simulink model "model"  (R2024a)
settings: Solver=FixedStepAuto  StartTime=0.0  StopTime=2500  FixedStep=0.01  RelTol=1e-3
values from neighbouring files (symbols this model uses):
  C_eq1 = [0.99 0 0 0 0 0 0 0 0 0 0 0 ... (924 elements, 22x42)]    [C_1.mat]
  C_eq2 = [0 0 0 0 0 0 0 0 0 0 0 0 ... (22 elements, 22x1)]    [C_2.mat]
  C_ineq1 = [0 0 0 0 0 0 0 0 0 0 0 0 ... (4704 elements, 112x42)]    [C_3.mat]
  C_ineq2 = [0.00443775952052 0.0171604689216 0.00443775952052 0.0171604689216 0.00443775952052 0.0171604689216 0.00443775952052 0.0171604689216 0.00443775952052 0.0171604689216 0.00443775952052 0.0171604689216 ... (112 elements, 112x1)]    [C_4.mat]
  H = [1 0 0 0 0 0 0 0 0 0 0 0 ... (1764 elements, 42x42)]    [H.mat]
settings Model: Creator=12911  LastModifiedBy=12911

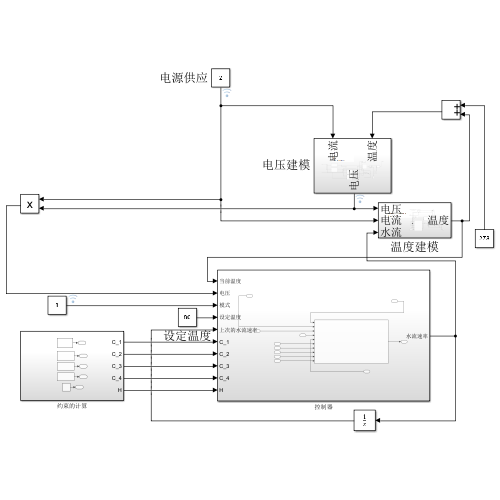
[thumbnail: Simulink's stored preview of the top-level diagram]
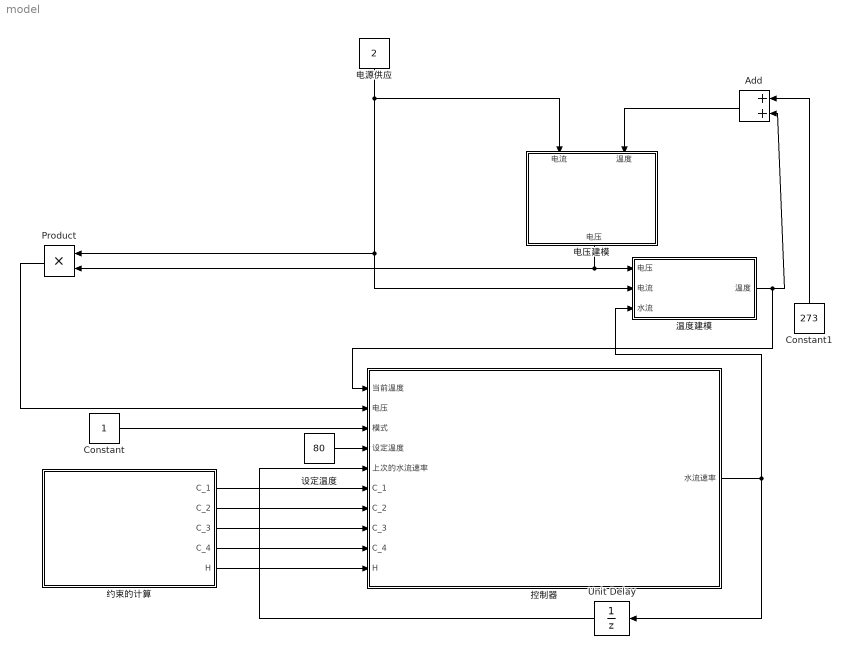
== system model ==
  Add : Sum
  Constant : Constant
  Constant1 : Constant  Value=273
  Product : Product
  Unit Delay : UnitDelay  SampleTime=-1  HasFrameUpgradeWarning=on
  控制器 : Subsystem
  温度建模 : Subsystem
  电压建模 : Subsystem
  电源供应 : Constant  Value=2
  约束的计算 : Subsystem
  设定温度 : Constant  Value=80
  wires:
  电源供应/1 -> 电压建模/1(电流), 温度建模/2(电流), Product/1
  电压建模/1(电压) -> Product/2, 温度建模/1(电压)
  Add/1 -> 电压建模/2(温度)
  Constant1/1 -> Add/1
  温度建模/1(温度) -> 控制器/1(当前温度), Add/2
  控制器/1(水流速率) -> 温度建模/3(水流), Unit Delay/1
  Product/1 -> 控制器/2(电压)
  Constant/1 -> 控制器/3(模式)
  设定温度/1 -> 控制器/4(设定温度)
  Unit Delay/1 -> 控制器/5(上次的水流速率)
  约束的计算/1(C_1) -> 控制器/6(C_1)
  约束的计算/2(C_2) -> 控制器/7(C_2)
  约束的计算/3(C_3) -> 控制器/8(C_3)
  约束的计算/4(C_4) -> 控制器/9(C_4)
  约束的计算/5(H) -> 控制器/10(H)

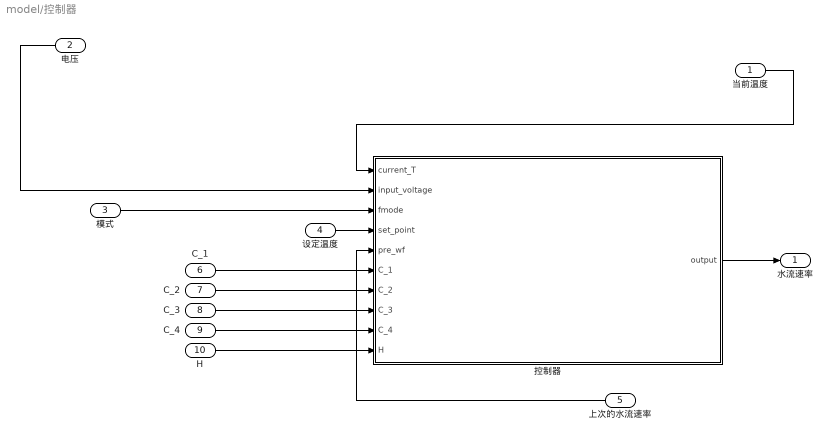
== system model/控制器 ==
  当前温度 : Inport
  电压 : Inport  Port=2
  模式 : Inport  Port=3
  设定温度 : Inport  Port=4
  上次的水流速率 : Inport  Port=5
  C_1 : Inport  Port=6
  C_2 : Inport  Port=7
  C_3 : Inport  Port=8
  C_4 : Inport  Port=9
  H : Inport  Port=10
  控制器 : MATLAB Function  TreatAsAtomicUnit=on
  水流速率 : Outport
  wires:
  当前温度/1 -> 控制器/1(current_T)
  H/1 -> 控制器/10(H)
  C_2/1 -> 控制器/7(C_2)
  模式/1 -> 控制器/3(fmode)
  C_3/1 -> 控制器/8(C_3)
  C_4/1 -> 控制器/9(C_4)
  上次的水流速率/1 -> 控制器/5(pre_wf)
  设定温度/1 -> 控制器/4(set_point)
  控制器/1(output) -> 水流速率/1
  电压/1 -> 控制器/2(input_voltage)
  C_1/1 -> 控制器/6(C_1)

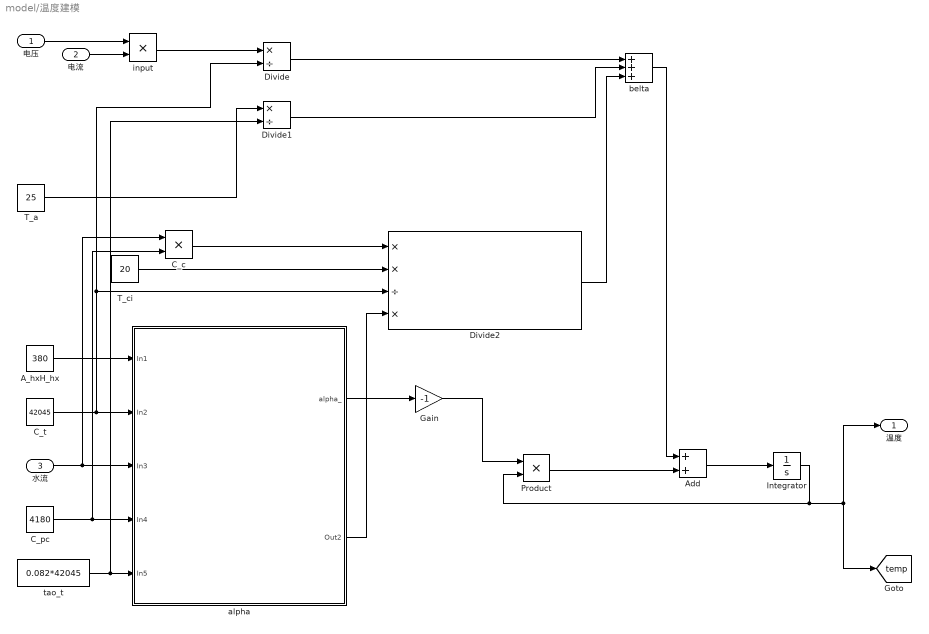
== system model/温度建模 ==
  电压 : Inport
  电流 : Inport  Port=2
  水流 : Inport  Port=3
  A_hxH_hx : Constant  Value=380
  Add : Sum
  C_c : Product
  C_pc : Constant  Value=4180
  C_t : Constant  Value=42045
  Divide : Product  Inputs=*/
  Divide1 : Product  Inputs=*/
  Divide2 : Product  Inputs=**/*
  Gain : Gain  Gain=-1
  Integrator : Integrator  InitialCondition=30
  Product : Product
  T_a : Constant  Value=25
  T_ci : Constant  Value=20
  alpha : Subsystem
  belta : Sum  Inputs=+++
  input : Product
  tao_t : Constant  Value=0.082*42045
  温度 : Outport
  tag scope: temp=global
  wires:
  电流/1 -> input/2
  电压/1 -> input/1
  A_hxH_hx/1 -> alpha/1(In1)
  C_t/1 -> Divide/2, Divide2/3, alpha/2(In2)
  水流/1 -> C_c/1, alpha/3(In3)
  C_pc/1 -> C_c/2, alpha/4(In4)
  tao_t/1 -> Divide1/2, alpha/5(In5)
  input/1 -> Divide/1
  T_a/1 -> Divide1/1
  Divide/1 -> belta/1
  Divide1/1 -> belta/2
  C_c/1 -> Divide2/1
  T_ci/1 -> Divide2/2
  alpha/2(Out2) -> Divide2/4
  Divide2/1 -> belta/3
  alpha/1(alpha_) -> Gain/1
  Gain/1 -> Product/1
  belta/1 -> Add/1
  Product/1 -> Add/2
  Add/1 -> Integrator/1
  Integrator/1 -> Product/2, 温度/1, [temp]

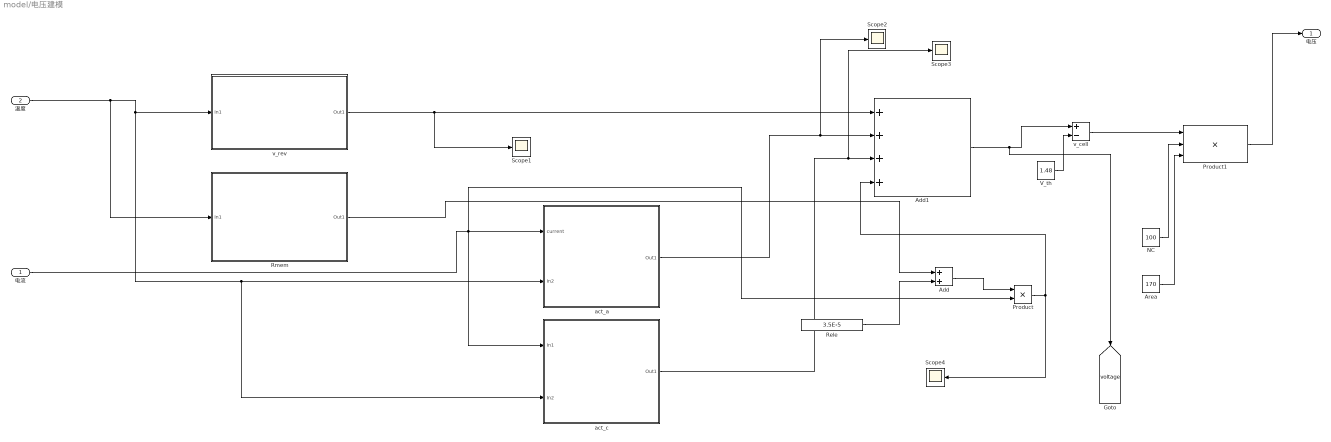
== system model/电压建模 ==
  电流 : Inport
  温度 : Inport  Port=2
  Add : Sum
  Add1 : Sum  Inputs=++++
  Area : Constant  Value=170
  NC : Constant  Value=100
  Product : Product
  Product1 : Product  Inputs=3
  Rele : Constant  Value=3.5E-5
  Rmem : Subsystem
  Scope{1..4} (4 alike) : Scope
  V_th : Constant  Value=1.48
  act_a : Subsystem
  act_c : Subsystem
  v_cell : Sum  Inputs=+-
  v_rev : Subsystem
  电压 : Outport
  tag scope: voltage=global
  wires:
  温度/1 -> Rmem/1(In1), act_c/2(In2), act_a/2(In2), v_rev/1(In1)
  v_rev/1(Out1) -> Scope1/1, Add1/1
  Rmem/1(Out1) -> Add/1
  Add1/1 -> [voltage], v_cell/1
  电流/1 -> act_c/1(In1), Product/2, act_a/1(current)
  act_a/1(Out1) -> Scope2/1, Add1/2
  act_c/1(Out1) -> Scope3/1, Add1/3
  Rele/1 -> Add/2
  Add/1 -> Product/1
  Product/1 -> Scope4/1, Add1/4
  V_th/1 -> v_cell/2
  v_cell/1 -> Product1/1
  NC/1 -> Product1/2
  Area/1 -> Product1/3
  Product1/1 -> 电压/1

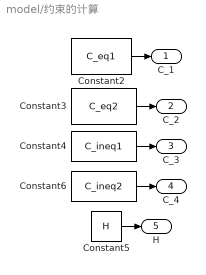
== system model/约束的计算 ==
  Constant2 : Constant  Value=C_eq1
  Constant3 : Constant  Value=C_eq2
  Constant4 : Constant  Value=C_ineq1
  Constant5 : Constant  Value=H
  Constant6 : Constant  Value=C_ineq2
  C_1 : Outport
  C_2 : Outport  Port=2
  C_3 : Outport  Port=3
  C_4 : Outport  Port=4
  H : Outport  Port=5
  wires:
  Constant4/1 -> C_3/1
  Constant6/1 -> C_4/1
  Constant2/1 -> C_1/1
  Constant5/1 -> H/1
  Constant3/1 -> C_2/1

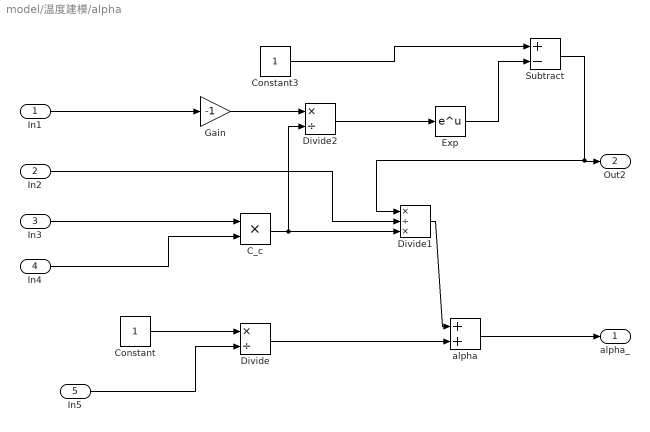
== system model/温度建模/alpha ==
  In1 : Inport
  In2 : Inport  Port=2
  In3 : Inport  Port=3
  In4 : Inport  Port=4
  In5 : Inport  Port=5
  C_c : Product
  Constant : Constant
  Constant3 : Constant
  Divide : Product  Inputs=*/
  Divide1 : Product  Inputs=*/*
  Divide2 : Product  Inputs=*/
  Exp : Math
  Gain : Gain  Gain=-1
  Subtract : Sum  Inputs=+-
  alpha : Sum
  alpha_ : Outport
  Out2 : Outport  Port=2
  wires:
  Constant/1 -> Divide/1
  Constant3/1 -> Subtract/1
  In1/1 -> Gain/1
  C_c/1 -> Divide1/3, Divide2/2
  Gain/1 -> Divide2/1
  Divide/1 -> alpha/2
  Exp/1 -> Subtract/2
  Divide2/1 -> Exp/1
  Subtract/1 -> Out2/1, Divide1/1
  Divide1/1 -> alpha/1
  In3/1 -> C_c/1
  alpha/1 -> alpha_/1
  In5/1 -> Divide/2
  In4/1 -> C_c/2
  In2/1 -> Divide1/2

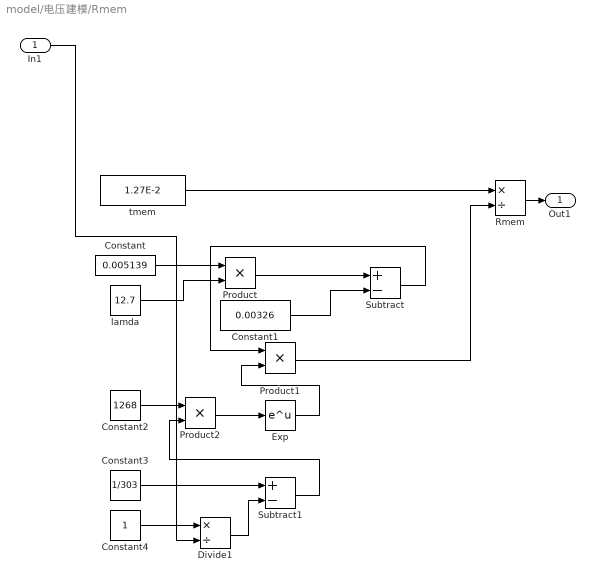
== system model/电压建模/Rmem ==
  In1 : Inport
  Constant : Constant  Value=0.005139
  Constant1 : Constant  Value=0.00326
  Constant2 : Constant  Value=1268
  Constant3 : Constant  Value=1/303
  Constant4 : Constant
  Divide1 : Product  Inputs=*/
  Exp : Math
  Product : Product
  Product1 : Product
  Product2 : Product
  Rmem : Product  Inputs=*/
  Subtract : Sum  Inputs=+-
  Subtract1 : Sum  Inputs=+-
  lamda : Constant  Value=12.7
  tmem : Constant  Value=1.27E-2
  Out1 : Outport
  wires:
  Product2/1 -> Exp/1
  Constant4/1 -> Divide1/1
  tmem/1 -> Rmem/1
  Exp/1 -> Product1/2
  Subtract/1 -> Product1/1
  Constant1/1 -> Subtract/2
  Subtract1/1 -> Product2/2
  lamda/1 -> Product/2
  Product1/1 -> Rmem/2
  Divide1/1 -> Subtract1/2
  Product/1 -> Subtract/1
  Constant2/1 -> Product2/1
  Constant/1 -> Product/1
  Constant3/1 -> Subtract1/1
  Rmem/1 -> Out1/1
  In1/1 -> Divide1/2

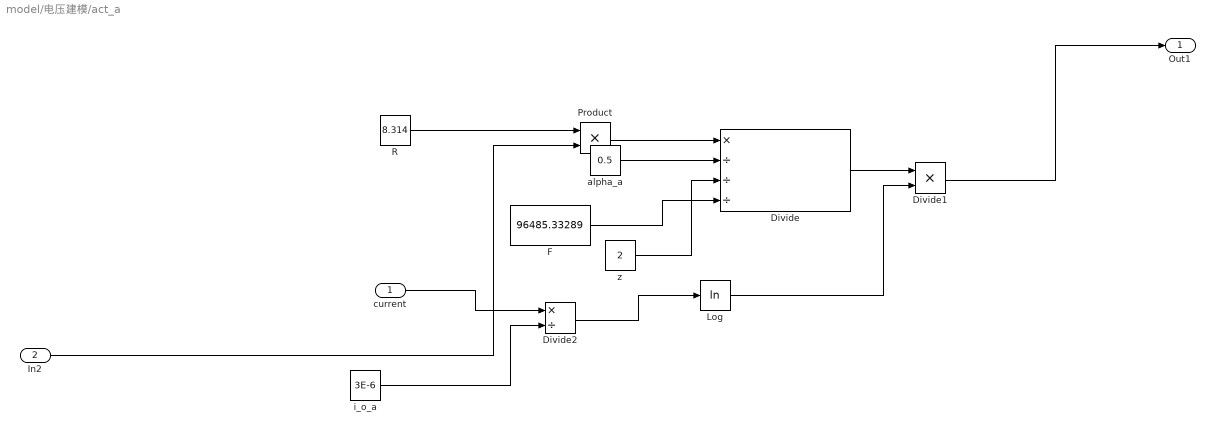
== system model/电压建模/act_a ==
  current : Inport
  In2 : Inport  Port=2
  Divide : Product  Inputs=*///
  Divide1 : Product  Inputs=**
  Divide2 : Product  Inputs=*/
  F : Constant  Value=96485.33289
  Log : Math  Operator=log
  Product : Product
  R : Constant  Value=8.314
  alpha_a : Constant  Value=0.5
  i_o_a : Constant  Value=3E-6
  z : Constant  Value=2
  Out1 : Outport
  wires:
  F/1 -> Divide/4
  i_o_a/1 -> Divide2/2
  Product/1 -> Divide/1
  z/1 -> Divide/3
  current/1 -> Divide2/1
  Divide2/1 -> Log/1
  Log/1 -> Divide1/2
  R/1 -> Product/1
  alpha_a/1 -> Divide/2
  Divide/1 -> Divide1/1
  Divide1/1 -> Out1/1
  In2/1 -> Product/2

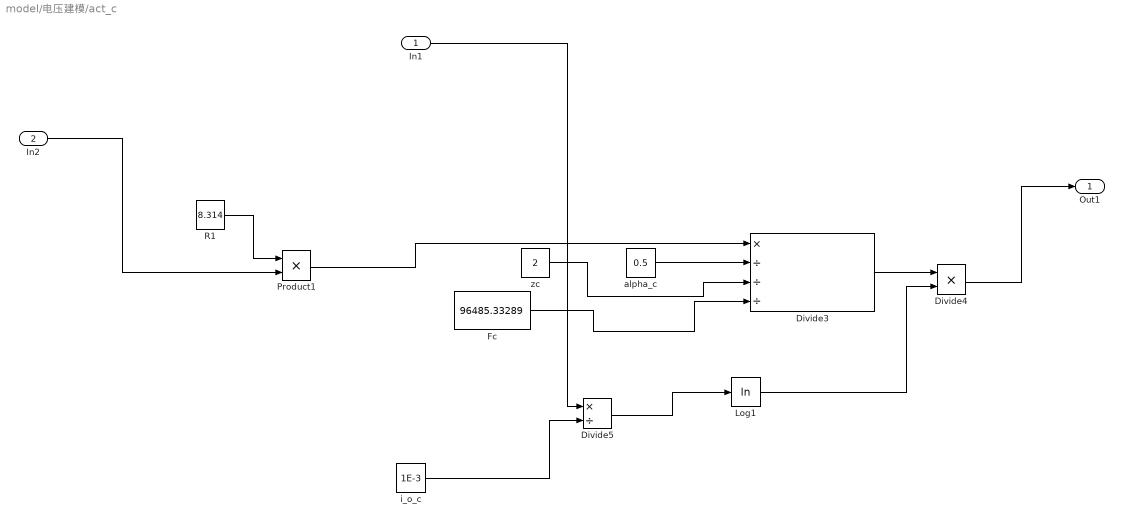
== system model/电压建模/act_c ==
  In1 : Inport
  In2 : Inport  Port=2
  Divide3 : Product  Inputs=*///
  Divide4 : Product  Inputs=**
  Divide5 : Product  Inputs=*/
  Fc : Constant  Value=96485.33289
  Log1 : Math  Operator=log
  Product1 : Product
  R1 : Constant  Value=8.314
  alpha_c : Constant  Value=0.5
  i_o_c : Constant  Value=1E-3
  zc : Constant  Value=2
  Out1 : Outport
  wires:
  Divide5/1 -> Log1/1
  Log1/1 -> Divide4/2
  Fc/1 -> Divide3/4
  alpha_c/1 -> Divide3/2
  R1/1 -> Product1/1
  i_o_c/1 -> Divide5/2
  zc/1 -> Divide3/3
  Product1/1 -> Divide3/1
  Divide3/1 -> Divide4/1
  Divide4/1 -> Out1/1
  In1/1 -> Divide5/1
  In2/1 -> Product1/2

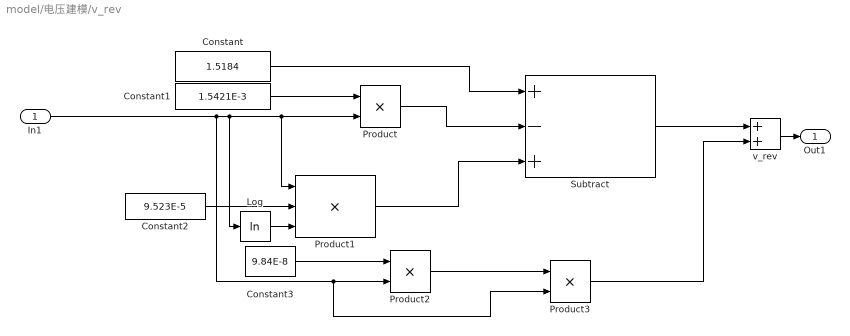
== system model/电压建模/v_rev ==
  In1 : Inport
  Constant : Constant  Value=1.5184
  Constant1 : Constant  Value=1.5421E-3
  Constant2 : Constant  Value=9.523E-5
  Constant3 : Constant  Value=9.84E-8
  Log : Math  Operator=log
  Product : Product
  Product1 : Product  Inputs=3
  Product2 : Product
  Product3 : Product
  Subtract : Sum  Inputs=+-+
  v_rev : Sum
  Out1 : Outport
  wires:
  Product/1 -> Subtract/2
  Constant3/1 -> Product2/1
  In1/1 -> Product/2, Product1/1, Log/1, Product3/2, Product2/2
  v_rev/1 -> Out1/1
  Product1/1 -> Subtract/3
  Product3/1 -> v_rev/2
  Constant2/1 -> Product1/2
  Constant/1 -> Subtract/1
  Log/1 -> Product1/3
  Constant1/1 -> Product/1
  Subtract/1 -> v_rev/1
  Product2/1 -> Product3/1

== matlab function model/控制器/控制器 ==
  data: current_T input; input_voltage input; fmode input; output output size=1*1; set_point input; pre_wf input; C_1 input; C_2 input; C_3 input; C_4 input; H input
function output = solduagwg(current_T,input_voltage, fmode,set_point,pre_wf,C_1,C_2,C_3,C_4,H)
         
    C_3 = C_3(41:end,:);
    C_4 = C_4(41:end,:);

    delta = 0.01;

    function y = solve_water_flow(current_T,input_voltage,constant,m_w,delta)
        C_t = 42045;
        C_pc = 4180;
        A_hxH_hx = 380;
        T_a = 25;
        T_ci = 20;
        tao_t = 0.082*42045;
        C_c_s = m_w*C_pc;
        alpha = 1/tao_t + (C_c_s/C_t)*(1-exp(-A_hxH_hx/C_c_s));
        belta = input_voltage/C_t + T_a/tao_t + (C_c_s*T_ci/C_t)*(1-exp(-A_hxH_hx/C_c_s));
        % aawinio = (-1/tao_t)*current_T+input(current_density)/C_t + T_a/tao_t;
        y = (-alpha*current_T+belta)*delta-constant;
    end
    
    function u = solve_MPC(current_x,C_1,C_2,C_3,C_4,H,fmode)
        B = [1 0;0 1]; 
        N_horizon = 10;
        Vold = zeros(size(B,1)*(N_horizon+1)+size(B,2)*N_horizon,fmode);
        idx_x0_start = 1;
        idx_x0_end = 2;

        C_eq1_init = zeros(2, 2*(10+1)+2*10);
        C_eq1_init(:, idx_x0_start:idx_x0_end) = eye(2);
        C_eq2_init = current_x;
        C_1 = [C_1;C_eq1_init];
        C_2 = [C_2;C_eq2_init];
        function [x_seq, u_seq,exitflag] = solve(Vold,C_1,C_2,C_3,C_4,H)
    
            options = optimoptions('quadprog','Algorithm','active-set');
            % options = optimoptions('quadprog', 'Display', 'none');
            x0 = zeros(42,1);
            % ws = optimwarmstart(x0,options);
            [var_optim, ~, exitflag] = quadprog(H, [], C_3, C_4, C_1, C_2, [], [], x0,options);
            if exitflag == -2
                var_optim = Vold;
            end
            % a = size(var_optim);
            % aduawgd  = var_optim(22);
            % xawudh = var_optim(1:2*(10+1),1);
            x_seq = reshape(var_optim(1:2*(10+1),1), 2, 10+1);
            u_seq = reshape(var_optim(2*(10+1)+1:42,1),2, 10);
        end
        [x_seq,u_seq,exitflag] = solve(Vold,C_1,C_2,C_3,C_4,H);
        u_nominal = u_seq(:, 1);
%             u_feedback_ = obj.sys.K * (x_init - x_nominal_seq(:, 1)); %改动
        u_feed = -0.01 * (current_x); 
        if fmode == 1
            u = u_nominal + u_feed;
        elseif fmode == 2
            u = u_feed;
        else
            u = u_nominal + u_feed;
        end
    end

    function [C_ineq1,C_ineq2] = add_UC_bond_ineq_constraint(UC_bond)
        C_ineq1 = [];
        C_ineq2 = [];
        min_v = UC_bond(1,2);
        max_v = UC_bond(1,1);
        
        G_add = [1 0;-1 0;0 1;0 -1];
        C_ineq2_add = [max_v;-min_v;max_v;-min_v];
        G_block = zeros(size(G_add,1),2*(10+1));
        for i=1:10
            G_U_block = [G_block,zeros(size(G_add,1),2*(i-1)),G_add,zeros(size(G_add,1),2*(10-i))];
            C_ineq1 = [C_ineq1;G_U_block];
            C_ineq2 = [C_ineq2;C_ineq2_add];
        end
    end

    u_feedback = -0.01*(current_T-set_point)*delta;
    bond = @(z)solve_water_flow(current_T,input_voltage,0,z,delta);

    UC_bond = [bond(0.0)-u_feedback,bond(1.0)-u_feedback];
    
    [c_UC_1,c_UC_2] = add_UC_bond_ineq_constraint(UC_bond);
    C_3 = [C_3;c_UC_1];
    C_4 = [C_4;c_UC_2];
    u = solve_MPC([current_T-set_point;current_T-set_point],C_1,C_2,C_3,C_4,H,fmode); %size(u) 2*1
    u = u(1,1);
    constant = u*delta;

    fun = @(z)solve_water_flow(current_T,input_voltage,constant,z,delta);

    if fun(1.0) <= 0 && fun(0.0) >= 0
        op = optimoptions('fsolve','Algorithm','levenberg-marquardt');
        output = fsolve(@(z)solve_water_flow(current_T,input_voltage,constant,z,delta),0.5,op);
    else
        output = pre_wf;
    end

end
